simulink model "simple_pwm"  (R2014a)
settings: Solver=VariableStepDiscrete  StartTime=0.0  StopTime=10.0  RelTol=1e-3
libraries: hdlsllib x1
settings Model: Creator=hirn.j  LastModifiedBy=hirn.j

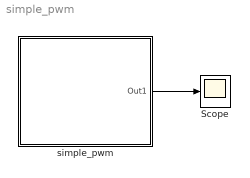
== system simple_pwm ==
  Scope : Scope
  simple_pwm : Subsystem
  wires:
  simple_pwm/1(Out1) -> Scope/1

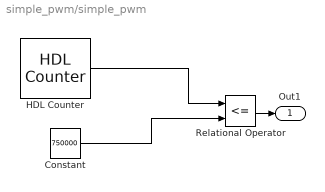
== system simple_pwm/simple_pwm ==
  Constant : Constant  Value=750000  OutDataTypeStr=uint32  SampleTime=1
  HDL Counter : hdlsllib/HDL Operations/HDL Counter  CountType=Count limited  CountInit=0  CountStep=1  CountMax=1000000  CountFromType=Initial value  CountFrom=0  CountResetPort=off  CountLoadPort=off  CountEnbPort=off  CountDirPort=off  CountDataType=Unsigned  CountWordLen=20  CountFracLen=0  CountSampTime=1
  Relational Operator : RelationalOperator  Operator=<=  OutDataTypeStr=boolean  SampleTime=1
  Out1 : Outport
  wires:
  Relational Operator/1 -> Out1/1
  HDL Counter/1 -> Relational Operator/1
  Constant/1 -> Relational Operator/2
